simulink subsystem "Vehicle1D_input_refsub"  (R2022a)
settings: Solver=VariableStepAuto  StartTime=0.0  StopTime=10.0  RelTol=1e-3
settings Model: Creator=isaacito  LastModifiedBy=isaacito

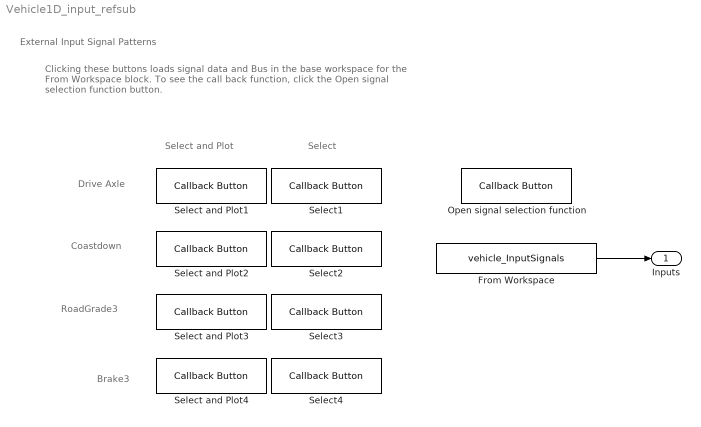
== system Vehicle1D_input_refsub ==
  note: Clicking these buttons loads signal data and Bus
      | in the base workspace for the From Workspace block.
      | To see the call back function,
      | click the Open signal selection function button.
  note: External Input Signal Patterns
  note: Drive Axle
  note: Coastdown
  note: RoadGrade3
  note: Brake3
  note: Select and Plot
  note: Select
  From Workspace : FromWorkspace  VariableName=vehicle_InputSignals  OutDataTypeStr=Bus: vehicle_InputBus  Interpolate=off  OutputAfterFinalValue=Holding final value
      settings: AttributesFormatString=|
      | %<OutDataTypeStr>
      | Interpolate: %<Interpolate>
  Open signal selection function : CallbackButton  ButtonText=Open function
      settings: ClickFcn=edit Vehicle1D_selectInput
  Select and Plot{1..4} (4 alike) : CallbackButton  ButtonText=Select and Plot
      Select and Plot1 settings: ClickFcn=|
      | Vehicle1D_selectInput( ...
      |     InputPattern = "DriveAxle", ...
      |     DisplayPlot = true, ...
      |     DisplayMessage = true )
      Select and Plot2 settings: ClickFcn=|
      | Vehicle1D_selectInput( ...
      |     InputPattern = "Coastdown", ...
      |     DisplayPlot = true, ...
      |     DisplayMessage = true )
      Select and Plot3 settings: ClickFcn=|
      | Vehicle1D_selectInput( ...
      |     InputPattern = "RoadGrade3", ...
      |     DisplayPlot = true, ...
      |     DisplayMessage = true )
      Select and Plot4 settings: ClickFcn=|
      | Vehicle1D_selectInput( ...
      |     InputPattern = "Brake3", ...
      |     DisplayPlot = true, ...
      |     DisplayMessage = true )
  Select{1..4} (4 alike) : CallbackButton  ButtonText=Select
      Select1 settings: ClickFcn=|
      | Vehicle1D_selectInput( ...
      |     InputPattern = "DriveAxle", ...
      |     DisplayMessage = true)
      Select2 settings: ClickFcn=|
      | Vehicle1D_selectInput( ...
      |     InputPattern = "Coastdown", ...
      |     DisplayMessage = true)
      Select3 settings: ClickFcn=|
      | Vehicle1D_selectInput( ...
      |     InputPattern = "RoadGrade3", ...
      |     DisplayMessage = true)
      Select4 settings: ClickFcn=|
      | Vehicle1D_selectInput( ...
      |     InputPattern = "Brake3", ...
      |     DisplayMessage = true)
  Inputs : Outport
  wires:
  From Workspace/1 -> Inputs/1
